simulink subsystem "ControlState_ref"  (R2021b)
settings: Solver=VariableStepAuto  StartTime=0.0  StopTime=10.0  RelTol=1e-3
settings Model: Creator=valen  LastModifiedBy=valen

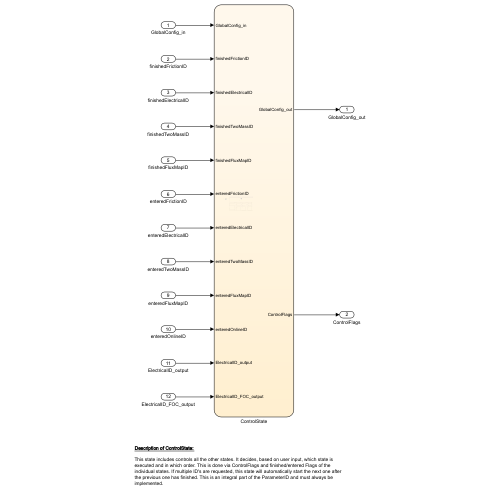
[thumbnail: Simulink's stored preview of the top-level diagram]
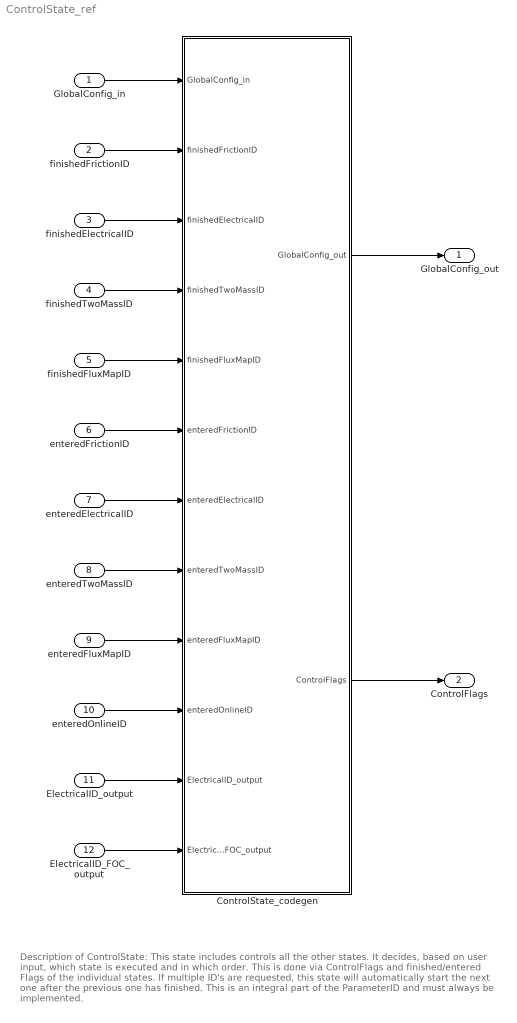
== system ControlState_ref ==
  note: Description of ControlState:
      |
      | This state includes controls all the other states. It decides, based on user input, which state is executed and in which order. This is done via ControlFlags and finished/entered Flags of the individual states. If multiple ID's are requested, this state will automatically start the next one after the previous one has finished. This is an integral part of the ParameterID and must always be implemented.
  GlobalConfig_in : Inport
  finishedFrictionID : Inport  Port=2
  finishedElectricalID : Inport  Port=3
  finishedTwoMassID : Inport  Port=4
  finishedFluxMapID : Inport  Port=5
  enteredFrictionID : Inport  Port=6
  enteredElectricalID : Inport  Port=7
  enteredTwoMassID : Inport  Port=8
  enteredFluxMapID : Inport  Port=9
  enteredOnlineID : Inport  Port=10
  ElectricalID_output : Inport  Port=11
  ElectricalID_FOC_output : Inport  Port=12
  ControlState_codegen : Stateflow chart  TreatAsAtomicUnit=on
      settings: PortSchema="{\"entries\":[{\"content\":{\"sides\":[{\"content\":{\"connectorIds\":[\"In11\",\"In1\",\"In2\",\"In3\",\"In4\",\"In5\",\"In8\",\"In7\",\"In6\",\"In12\",\"In9\",\"In10\"]},\"type\":\"ConnectorPlacement.EquallySpacedRectSide\",\"uuid\":\"3338e9a8-28b4-45bb-be16-581ebbf0e7d5\"},{\"content\":{\"connectorIds\":[\"Out1\",\"Out2\"],\"side\":\"RIGHT\"},\"type\":\"ConnectorPlacement.EquallySpacedRectSide\",\"uuid\":\"68ffdf0a-d88e-422d-a36e-256c991e1a1a\"},{\"content\":{\"connectorIds\":[],\"side\":\"TOP\"},\"type\":\"ConnectorPlacement.EquallySpacedRectSide\",\"uuid\":\"571bf6fb-233c-470d-b735-d23e4cf83e69\"}]},\"type\":\"ConnectorPlacement.EquallySpacedConnector\",\"uuid\":\"829c5db0-50d3-4caf-9d4e-ee907b3905d4\"}],\"packageUris\":[\"http://schema.mathworks.com/mf0/Connector/R2020b\"],\"version\":\"1.0\"}"
  GlobalConfig_out : Outport
  ControlFlags : Outport  Port=2
  wires:
  enteredOnlineID/1 -> ControlState_codegen/12(enteredOnlineID)
  GlobalConfig_in/1 -> ControlState_codegen/11(GlobalConfig_in)
  ControlState_codegen/1(GlobalConfig_out) -> GlobalConfig_out/1
  ElectricalID_output/1 -> ControlState_codegen/9(ElectricalID_output)
  finishedFluxMapID/1 -> ControlState_codegen/4(finishedFluxMapID)
  ElectricalID_FOC_output/1 -> ControlState_codegen/10(ElectricalID_FOC_output)
  ControlState_codegen/2(ControlFlags) -> ControlFlags/1
  finishedElectricalID/1 -> ControlState_codegen/2(finishedElectricalID)
  enteredFrictionID/1 -> ControlState_codegen/5(enteredFrictionID)
  enteredTwoMassID/1 -> ControlState_codegen/7(enteredTwoMassID)
  enteredElectricalID/1 -> ControlState_codegen/8(enteredElectricalID)
  finishedFrictionID/1 -> ControlState_codegen/1(finishedFrictionID)
  enteredFluxMapID/1 -> ControlState_codegen/6(enteredFluxMapID)
  finishedTwoMassID/1 -> ControlState_codegen/3(finishedTwoMassID)

== stateflow chart ControlState_ref/ControlState_codegen ==
  settings: updateMethod=DISCRETE  sampleTime=1/d_f_states
  note: ControlState
  state ControlState
    entry:
    during:
    GlobalConfig_out.Reset = GlobalConfig_in.Reset;
    GlobalConfig_out.ACCEPT = GlobalConfig_in.ACCEPT;
    GlobalConfig_out.enableParameterID = GlobalConfig_in.enableParameterID;
    GlobalConfig_out.ElectricalID = GlobalConfig_in.ElectricalID;
    GlobalConfig_out.FrictionID = GlobalConfig_in.FrictionID
    GlobalConfig_out.TwoMassID = GlobalConfig_in.TwoMassID;
    GlobalConfig_out.FluxMapID = GlobalConfig_in.FluxMapID;
    GlobalConfig_out.OnlineID = GlobalConfig_in.OnlineID;
    GlobalConfig_out.sampleTimeISR = GlobalConfig_in.sampleTimeISR;
    state decideMotorID
      entry:
      during:
      if (GlobalConfig_in.ACCEPT == 1)
      decideIDstates;
      end
      if(ControlFlags.finished_all_Offline_states == 1 && GlobalConfig_in.OnlineID==1 && enteredOnlineID==0)
      ControlFlags.enableOnlineID=boolean(1);
      elseif (ControlFlags.finished_all_Offline_states == 1 && GlobalConfig_in.OnlineID==0 && enteredOnlineID==1)
      ControlFlags.enableOnlineID=boolean(0);
      end
      exit:
    state activateFrictionID
      entry:
      ControlFlags.startFrictionID=boolean(1);
      during:
      exit:
    state activateFluxMapID
      entry:
      ControlFlags.startFluxMapID=boolean(1);
      during:
      exit:
    state activateTwoMassID
      entry:
      ControlFlags.startTwoMassID=boolean(1);
      during:
      exit:
    state activateElectricalID
      entry:
      ControlFlags.startElectricalID=boolean(1);
      during:
      exit:
    state duringElectricalID
      entry:
      ControlFlags.startElectricalID=boolean(0);
      during:
      GlobalConfig_out.PMSM_config.Ld_Henry=ElectricalID_output.PMSM_parameters.Ld_Henry;
      GlobalConfig_out.PMSM_config.Lq_Henry=ElectricalID_output.PMSM_parameters.Lq_Henry;
      GlobalConfig_out.PMSM_config.R_ph_Ohm=ElectricalID_output.PMSM_parameters.R_ph_Ohm;
      GlobalConfig_out.PMSM_config.Psi_PM_Vs=ElectricalID_output.PMSM_parameters.Psi_PM_Vs;
      GlobalConfig_out.PMSM_config.polePairs=ElectricalID_output.PMSM_parameters.polePairs;
      GlobalConfig_out.PMSM_config.J_kg_m_squared=....
      ElectricalID_output.PMSM_parameters.J_kg_m_squared;
      GlobalConfig_out.Kp_id=ElectricalID_FOC_output.Kp_id_out;
      GlobalConfig_out.Kp_iq=ElectricalID_FOC_output.Kp_iq_out;
      GlobalConfig_out.Kp_n=ElectricalID_FOC_output.Kp_n_out;
      GlobalConfig_out.Ki_id=ElectricalID_FOC_output.Ki_id_out;
      GlobalConfig_out.Ki_iq=ElectricalID_FOC_output.Ki_iq_out;
      GlobalConfig_out.Ki_n=ElectricalID_FOC_output.Ki_n_out;
      GlobalConfig_out.PMSM_6ph_inductances = ElectricalID_output.inductances_6ph;
      exit:
    state duringTwoMassID
      entry:
      ControlFlags.startTwoMassID=boolean(0);
      during:
      exit:
    state duringFrictionID
      entry:
      ControlFlags.startFrictionID=boolean(0);
      during:
      exit:
    state duringFluxMapID
      entry:
      ControlFlags.startFluxMapID=boolean(0);
      during:
      exit:
    state finishedFrictionID
      entry:
      finishedFrictionID_loc=uint16(2);
      during:
      exit:
      ControlFlags.transNr=uint16(0);
    state finishedFluxMapID
      entry:
      finishedFluxMapID_loc=uint16(2);
      during:
      exit:
      ControlFlags.transNr=uint16(0);
    state finishedTwoMassID
      entry:
      finishedTwoMassID_loc=uint16(2);
      during:
      exit:
      ControlFlags.transNr=uint16(0);
    state finishedElectricalID
      entry:
      finishedElectricalID_loc=uint16(2);
      during:
      exit:
      ControlFlags.transNr=uint16(0);
    (default) -> decideMotorID
    decideMotorID -> activateElectricalID [order 1] : [ControlFlags.transNr==1 && finishedElectricalID_loc==0]
    activateElectricalID -> decideMotorID [order 2] : [GlobalConfig_in.ElectricalID==0]
        | {ControlFlags.transNr = 0}
    duringElectricalID -> decideMotorID [order 2] : [GlobalConfig_in.ElectricalID==0]
        | {ControlFlags.transNr = 0}
    finishedElectricalID -> decideMotorID
    finishedTwoMassID -> decideMotorID
    decideMotorID -> activateTwoMassID [order 3] : [ControlFlags.transNr==2 && finishedTwoMassID_loc==0]
    activateTwoMassID -> decideMotorID [order 2] : [GlobalConfig_in.TwoMassID==0]
        | {ControlFlags.transNr = 0}
    duringTwoMassID -> decideMotorID [order 2] : [GlobalConfig_in.TwoMassID==0]
        | {ControlFlags.transNr = 0}
    finishedFrictionID -> decideMotorID
    decideMotorID -> activateFrictionID [order 4] : [ControlFlags.transNr==3 && finishedFrictionID_loc==0]
    activateFrictionID -> decideMotorID [order 2] : [GlobalConfig_in.FrictionID==0]
        | {ControlFlags.transNr = 0}
    duringFrictionID -> decideMotorID [order 2] : [GlobalConfig_in.FrictionID==0]
        | {ControlFlags.transNr = 0}
    finishedFluxMapID -> decideMotorID
    decideMotorID -> activateFluxMapID [order 2] : [ControlFlags.transNr==4 && finishedFluxMapID_loc==0]
    activateFluxMapID -> decideMotorID [order 2] : [GlobalConfig_in.FluxMapID==0]
        | {ControlFlags.transNr = 0}
    duringFluxMapID -> decideMotorID [order 2] : [GlobalConfig_in.FluxMapID==0]
        | {ControlFlags.transNr = 0}
    activateElectricalID -> duringElectricalID [order 1] : [enteredElectricalID==1]
    activateTwoMassID -> duringTwoMassID [order 1] : [enteredTwoMassID==1]
    activateFrictionID -> duringFrictionID [order 1] : [enteredFrictionID==1]
    activateFluxMapID -> duringFluxMapID [order 1] : [enteredFluxMapID==1]
    duringTwoMassID -> finishedTwoMassID [order 1] : [finishedTwoMassID==1]
    duringFrictionID -> finishedFrictionID [order 1] : [finishedFrictionID==1]
    duringFluxMapID -> finishedFluxMapID [order 1] : [finishedFluxMapID==1]
    duringElectricalID -> finishedElectricalID [order 1] : [finishedElectricalID==1]
  state Waiting
    entry:
    initParams;
    %wait for activation of
    %FrictionID
    %donothing
  note: ---
  Waiting -> ControlState [order 1] : [GlobalConfig_in.enableParameterID==1 && ....
      | GlobalConfig_in.Reset==0]
  (default) -> Waiting
  ControlState -> Waiting : [GlobalConfig_in.Reset==1 ||....
      |  GlobalConfig_in.enableParameterID==0]
  Waiting -> Waiting [order 2] : [GlobalConfig_in.Reset==1]
  data: finishedFrictionID input boolean; finishedElectricalID input boolean; finishedTwoMassID input boolean; finishedFluxMapID input boolean; enteredFrictionID input boolean; enteredFluxMapID input boolean; enteredTwoMassID input boolean; enteredElectricalID input boolean; ElectricalID_output input Bus: uz_ParaID_ElectricalID_output_t; finishedElectricalID_loc local; finishedFrictionID_loc local; finishedTwoMassID_loc local; finishedFluxMapID_loc local; ElectricalID_FOC_output input Bus: uz_ParaID_Controller_Parameters_output_t; GlobalConfig_in input Bus: uz_ParaID_GlobalConfig_t; GlobalConfig_out output Bus: uz_ParaID_GlobalConfig_t; ControlFlags output Bus: uz_ParaID_ControlFlags_t; enteredOnlineID input
  function decideIDstates:
    | function decideIDstates
    | %If the specific Identification Part is not selected (==0), treat it, as if
    | %it has finished
    | if(GlobalConfig_in.ElectricalID==0)
    |     finishedElectricalID_loc=uint16(1);
    | elseif(finishedElectricalID==1)
    |     finishedElectricalID_loc=uint16(2);
    | end
    | 
    | if(GlobalConfig_in.FrictionID==0)
    |     finishedFrictionID_loc=uint16(1);
    | elseif(finishedFrictionID==1)
    |      finishedFrictionID_loc=uint16(2);
    | end
    | 
    | if(GlobalConfig_in.TwoMassID==0)
    |     finishedTwoMassID_loc=uint16(1);
    | elseif(finishedTwoMassID==1)
    |     finishedTwoMassID_loc=uint16(2);
    | end
    | 
    | if(GlobalConfig_in.FluxMapID==0)
    |     finishedFluxMapID_loc=uint16(1);
    | elseif(finishedFluxMapID==1)
    |     finishedFluxMapID_loc=uint16(2);    
    | end
    | 
    | if(ControlFlags.finished_all_Offline_states == 0)
    |     %Determine path through the ElectricalID-Stateflows
    |     if(GlobalConfig_in.ElectricalID==1 && enteredElectricalID==0 && finishedElectricalID_loc~=2 && finishedElectricalID==0)
    |             ControlFlags.transNr=uint16(1);
    |             finishedElectricalID_loc = uint16(0);
    |     end
    | 
    |     %Determine path through the TwoMassID-Stateflows
    |     if(GlobalConfig_in.TwoMassID==1 && enteredTwoMassID==0 && finishedElectricalID_loc~=0 && finishedTwoMassID_loc~=2 && finishedTwoMassID==0)
    |             ControlFlags.transNr=uint16(2);
    |             finishedTwoMassID_loc = uint16(0);
    |     end
    |     
    |     %Determine path through the FrictionID-Stateflows
    |     if(GlobalConfig_in.FrictionID==1 && enteredFrictionID==0 && finishedElectricalID_loc~=0....
    |        && finishedTwoMassID_loc~=0 && finishedFrictionID_loc~=2 && finishedFrictionID==0)
    |            ControlFlags.transNr=uint16(3);
    |            finishedFrictionID_loc = uint16(0);
    |     end
    | 
    |     %Determine path through the FluxMapID-Stateflows
    |     if(GlobalConfig_in.FluxMapID==1 && enteredFluxMapID==0 && finishedElectricalID_loc~=0....
    |       && finishedTwoMassID_loc~=0 && finishedFrictionID_loc~=0 && finishedFluxMapID_loc~=2 && finishedFluxMapID==0)
    |             ControlFlags.transNr=uint16(4);
    |             finishedFluxMapID_loc = uint16(0);
    |     end
    | end
    | 
    | if(finishedElectricalID_loc~=0 && finishedTwoMassID_loc~=0 && ....
    |         finishedFrictionID_loc~=0 && finishedFluxMapID_loc~=0)
    |     ControlFlags.finished_all_Offline_states = boolean(1);
    | end
    | 
    | end
  function initParams:
    | function initParams
    | %Initialize Variables
    | finishedElectricalID_loc=uint16(0);
    | finishedFrictionID_loc=uint16(0);
    | finishedTwoMassID_loc=uint16(0);
    | finishedFluxMapID_loc=uint16(0);
    | 
    | %Initialize Outputs
    | ControlFlags.startFrictionID             = boolean(0);
    | ControlFlags.startElectricalID           = boolean(0);
    | ControlFlags.startTwoMassID              = boolean(0);
    | ControlFlags.startFluxMapID              = boolean(0);
    | GlobalConfig_out                         = GlobalConfig_in;
    | ControlFlags.enableOnlineID              = boolean(0);
    | ControlFlags.transNr                     = uint16(0);
    | ControlFlags.finished_all_Offline_states = boolean(0);
    | end
